simulink model "cluster_robot_control_6_moving_xd"  (R2016a)
settings: Solver=VariableStepAuto  StartTime=0.0  StopTime=30  RelTol=1e-3
values from neighbouring files (symbols this model uses):
  E = eye(8)    [cluster_robot_control_7_rotation.m]    (also in cluster_robot_control_8_final.m)
  LK1 = -LK1    [cluster_robot_control_7_rotation.m]    (also in cluster_robot_control_8_final.m)
  v0 = [1 1 2 1 1 1 1 1]'    [cluster_robot_control_7_rotation.m]    (also in cluster_robot_control_8_final.m)
  x0 = [1 3 2 1 3 2 4 5]'    [cluster_robot_control_7_rotation.m]    (also in cluster_robot_control_8_final.m)
  xd = [0 0 0 0 0 0 0 0]    [cluster_robot_control_7_rotation.m]    (also in cluster_robot_control_8_final.m)
settings Model: Creator=richa  LastModifiedBy=richa

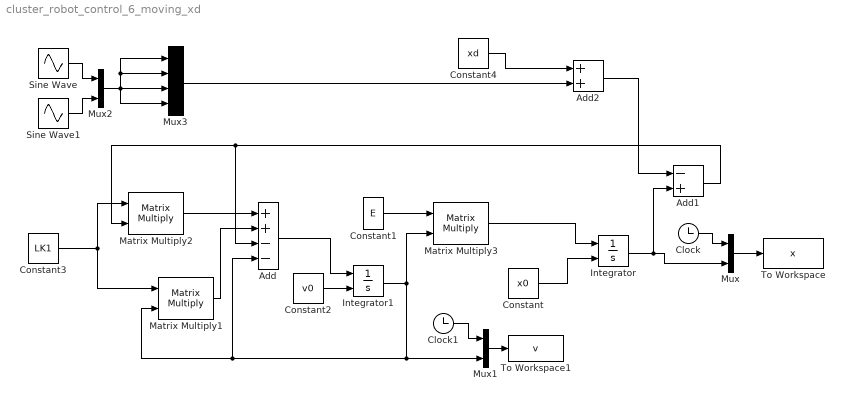
== system cluster_robot_control_6_moving_xd ==
  Add : Sum  Inputs=++--
  Add1 : Sum  Inputs=-+
  Add2 : Sum
  Clock : Clock
  Clock1 : Clock
  Constant : Constant  Value=x0
  Constant1 : Constant  Value=E
  Constant2 : Constant  Value=v0
  Constant3 : Constant  Value=LK1
  Constant4 : Constant  Value=xd
  Integrator : Integrator  InitialConditionSource=external
  Integrator1 : Integrator  InitialConditionSource=external
  Matrix Multiply1 : Product  Multiplication=Matrix(*)
  Matrix Multiply2 : Product  Multiplication=Matrix(*)
  Matrix Multiply3 : Product  Multiplication=Matrix(*)
  Mux : Mux  Inputs=2
  Mux1 : Mux  Inputs=2
  Mux2 : Mux  Inputs=2
  Mux3 : Mux
  Sine Wave : Sin  Amplitude=100  SampleTime=0
  Sine Wave1 : Sin  Amplitude=100  Phase=pi/2  SampleTime=0
  To Workspace : ToWorkspace  VariableName=x  SampleTime=-1
  To Workspace1 : ToWorkspace  VariableName=v  SampleTime=-1
  wires:
  Constant/1 -> Integrator/2
  Mux/1 -> To Workspace/1
  Clock/1 -> Mux/1
  Constant2/1 -> Integrator1/2
  Constant3/1 -> Matrix Multiply1/1, Matrix Multiply2/1
  Mux1/1 -> To Workspace1/1
  Clock1/1 -> Mux1/1
  Matrix Multiply2/1 -> Add/1
  Matrix Multiply1/1 -> Add/2
  Add/1 -> Integrator1/1
  Constant1/1 -> Matrix Multiply3/1
  Matrix Multiply3/1 -> Integrator/1
  Add1/1 -> Add/3, Matrix Multiply2/2
  Integrator/1 -> Add1/2, Mux/2
  Integrator1/1 -> Matrix Multiply3/2, Matrix Multiply1/2, Add/4, Mux1/2
  Sine Wave/1 -> Mux2/1
  Sine Wave1/1 -> Mux2/2
  Mux2/1 -> Mux3/1, Mux3/2, Mux3/3, Mux3/4
  Constant4/1 -> Add2/1
  Mux3/1 -> Add2/2
  Add2/1 -> Add1/1
